simulink model "generic_IVS"  (R2024a)
settings: Solver=FixedStepDiscrete  StartTime=0.0  StopTime=inf  FixedStep=0.001  RelTol=1e-3
undefined symbols (not defined in the file): do_waypoints_tail_shifted_2, global_path_xy_second_test, pathXY, route1_waypoint, route1_waypoint_raw, route2_waypoint, route2_waypoint_raw, route3_waypoint, route3_waypoint_raw
libraries: CarMaker4SL x134, slpidlib x4, simulink x1
(part 5 of 5)

== matlab function generic_IVS/CarMaker/Subsystem/Final Project/Scenario 1/MATLAB Function ==
  settings: updateMethod=DISCRETE  sampleTime=1.0
  data: waypoints input; startIdx input; global_path_xy_dense output; must1 input; must2 input; goalIdx input; state input
% function global_path_xy_dense = make_global_path(waypoints, startIdx, must1, must2, goalIdx)
% %#codegen
% 
% N = size(waypoints,1);
% max_neighbors = 20;
% MAXLEN = 2000; % 충분히 크게
% 
% % --- via_nodes 처리 ---
% via_nodes = startIdx;
% if must1 ~= 0
%     via_nodes = [via_nodes, must1];
% end
% if must2 ~= 0
%     via_nodes = [via_nodes, must2];
% end
% via_nodes = [via_nodes, goalIdx];
% 
% % --- 진행방향 단위 벡터 계산 ---
% forward_vecs = zeros(N,2);
% for i = 1:N-1
%     v = waypoints(i+1,:) - waypoints(i,:);
%     vn = norm(v);
%     if vn > 1e-6
%         forward_vecs(i,:) = v / vn;
%     else
%         forward_vecs(i,:) = [1,0];
%     end
% end
% forward_vecs(N,:) = forward_vecs(N-1,:);
% 
% % --- 이웃 리스트 (고정 double array) ---
% neighborList = zeros(N, max_neighbors);
% neighborNum  = zeros(N,1);
% D_thresh = 5;
% 
% for i = 1:N
%     dists = sqrt(sum((waypoints - waypoints(i,:)).^2, 2));
%     candidateIdx = find(dists > 0 & dists < D_thresh);
% ncnt = 0;
% for j = 1:length(candidateIdx)
%     idx = candidateIdx(j);
%     vec = waypoints(idx,:) - waypoints(i,:);
%     vn2 = norm(vec);
%     if vn2 < 1e-6
%         continue;
%     end
%     vec = vec / vn2;
%     if dot(forward_vecs(i,:), vec) > 0
%         if ncnt < max_neighbors   % <--- 바꿔주세요!
%             ncnt = ncnt+1;
%             neighborList(i,ncnt) = idx;
%         end
%     end
% end
% neighborNum(i) = ncnt;
% end
% 
% % --- 전체 경로 연결 (via_nodes 순서대로, preallocation) ---
% full_path = zeros(N * (length(via_nodes)-1), 1);
% full_idx = 1;
% 
% for seg = 1:(length(via_nodes)-1)
%     sIdx = via_nodes(seg);
%     gIdx = via_nodes(seg+1);
% 
%     cameFrom = zeros(N,1);
%     gScore   = inf(N,1);
%     fScore   = inf(N,1);
% 
%     gScore(sIdx) = 0;
%     fScore(sIdx) = norm(waypoints(sIdx,:) - waypoints(gIdx,:));
%     openSet = zeros(N,1);
%     openSet(1) = sIdx;
%     openLen = 1;
% 
%     found = false;
%     while openLen > 0
%         fvalues = zeros(openLen,1);
%         for i = 1:openLen
%             fvalues(i) = fScore(openSet(i));
%         end
%         [~, minIdx] = min(fvalues);
%         current = openSet(minIdx);
%         if current == gIdx
%             found = true;
%             break;
%         end
%         if minIdx < openLen
%             openSet(minIdx:openLen-1) = openSet(minIdx+1:openLen);
%         end
%         openLen = openLen - 1;
% 
%         for nidx = 1:neighborNum(current)
%             neighbor = neighborList(current, nidx);
%             edge_cost = norm(waypoints(neighbor,:) - waypoints(current,:));
%             tentative_gScore = gScore(current) + edge_cost;
%             if tentative_gScore < gScore(neighbor)
%                 cameFrom(neighbor) = current;
%                 gScore(neighbor)   = tentative_gScore;
%                 fScore(neighbor)   = tentative_gScore + norm(waypoints(neighbor,:) - waypoints(gIdx,:));
%                 isin = false;
%                 for q = 1:openLen
%                     if openSet(q) == neighbor
%                         isin = true;
%                         break;
%                     end
%                 end
%                 if ~isin && openLen < N
%                     openLen = openLen+1;
%                     openSet(openLen) = neighbor;
%                 end
%             end
%         end
%     end
% 
%     if ~found
%         global_path_xy_dense = zeros(MAXLEN,2); % error 방지
%         return
%     end
% 
%     % --- 경로 추적 (preallocation) ---
%     MAX_PATH_LEN = N;
%     tmp_path = zeros(MAX_PATH_LEN, 1);
%     idx = 1;
%     curr = gIdx;
%     while curr ~= sIdx
%         tmp_path(idx) = curr;
%         curr = cameFrom(curr);
%         idx = idx + 1;
%         if idx > MAX_PATH_LEN
%             break;
%         end
%     end
%     tmp_path(idx) = sIdx;
%     path = tmp_path(idx:-1:1);
% 
%     if seg > 1
%         path = path(2:end);
%     end
% 
%     lenp = length(path);
%     full_path(full_idx : full_idx+lenp-1) = path;
%     full_idx = full_idx + lenp;
% end
% 
% full_path = full_path(1:full_idx-1);
% 
% % --- 경로 좌표 추출 ---
% global_path_xy = waypoints(full_path, :);
% 
% % --- 보간을 통한 촘촘한 경로 생성 ---
% diffs = diff(global_path_xy);
% seg_len = sqrt(sum(diffs.^2, 2));
% s = [0; cumsum(seg_len)];
% ds_interp = 0.5;
% if s(end) < ds_interp
%     interp_xy = global_path_xy;
% else
%     s_interp = (0:ds_interp:s(end))';
%     x_interp = interp1(s, global_path_xy(:,1), s_interp, 'linear');
%     y_interp = interp1(s, global_path_xy(:,2), s_interp, 'linear');
%     interp_xy = [x_interp, y_interp];
% end
% 
% global_path_xy_dense = zeros(MAXLEN,2);
% real_len = size(interp_xy,1);
% if real_len > MAXLEN
%     real_len = MAXLEN;
% end
% global_path_xy_dense(1:real_len,:) = interp_xy(1:real_len,:);
% end


function global_path_xy_dense = make_global_path_with_fsm_sfunc(waypoints, startIdx, must1, must2, goalIdx, state)
% Simulink에서 사용할 수 있도록 만든 FSM 기반 global path 생성 함수
% 입력:
%   waypoints [Nx2] double, startIdx/must1/must2/goalIdx/state: double scalar
% 출력:
%   global_path_xy_dense [MAXLEN x 2] double

%#codegen

MAXLEN = 2000;
N = size(waypoints,1);

persistent prev_goalIdx prev_full_path prev_flag

if isempty(prev_goalIdx)
    prev_goalIdx = goalIdx;
end
if isempty(prev_flag)
    prev_flag = 1; % default값. 반드시 0,1로만 동작
end

% Simulink 실행 시마다 state=0에서 "한 번만" 새 경로 생성
if state == 0
    startIdx_new = prev_goalIdx;
    must1_new = 0;
    must2_new = 0;
    goalIdx_new = 1565;

    % prev_flag가 1→0으로 바뀌는 순간 한 번만 실행
    if prev_flag ~= 0
        global_path_xy_dense = gen_global_path(waypoints, startIdx_new, must1_new, must2_new, goalIdx_new, N, MAXLEN);
        prev_full_path = global_path_xy_dense;
        prev_goalIdx = goalIdx_new;
    else
        % 이미 만든 경로 유지
        if isempty(prev_full_path)
            global_path_xy_dense = zeros(MAXLEN,2);
        else
            global_path_xy_dense = prev_full_path;
        end
    end
    prev_flag = 0;
else % state==1
    global_path_xy_dense = gen_global_path(waypoints, startIdx, must1, must2, goalIdx, N, MAXLEN);
    prev_full_path = global_path_xy_dense;
    prev_goalIdx = goalIdx;
    prev_flag = 1;
end

end

% ---- 내부 subfunction ----
function global_path_xy_dense = gen_global_path(waypoints, startIdx, must1, must2, goalIdx, N, MAXLEN)

max_neighbors = 20;
% --- via_nodes 처리 ---
via_nodes = startIdx;
if must1 ~= 0
    via_nodes = [via_nodes, must1];
end
if must2 ~= 0
    via_nodes = [via_nodes, must2];
end
via_nodes = [via_nodes, goalIdx];

% --- 진행방향 단위 벡터 계산 ---
forward_vecs = zeros(N,2);
for i = 1:N-1
    v = waypoints(i+1,:) - waypoints(i,:);
    vn = norm(v);
    if vn > 1e-6
        forward_vecs(i,:) = v / vn;
    else
        forward_vecs(i,:) = [1,0];
    end
end
forward_vecs(N,:) = forward_vecs(N-1,:);

% --- 이웃 리스트 ---
neighborList = zeros(N, max_neighbors);
neighborNum  = zeros(N,1);
D_thresh = 5;

for i = 1:N
    dists = sqrt(sum((waypoints - waypoints(i,:)).^2, 2));
    candidateIdx = find(dists > 0 & dists < D_thresh);
    ncnt = 0;
    for j = 1:length(candidateIdx)
        idx = candidateIdx(j);
        vec = waypoints(idx,:) - waypoints(i,:);
        vn2 = norm(vec);
        if vn2 < 1e-6
            continue;
        end
        vec = vec / vn2;
        if dot(forward_vecs(i,:), vec) > 0
            if ncnt < max_neighbors
                ncnt = ncnt+1;
                neighborList(i,ncnt) = idx;
            end
        end
    end
    neighborNum(i) = ncnt;
end

% --- 전체 경로 연결 (via_nodes 순서대로, preallocation) ---
full_path = zeros(N * (length(via_nodes)-1), 1);
full_idx = 1;

for seg = 1:(length(via_nodes)-1)
    sIdx = via_nodes(seg);
    gIdx = via_nodes(seg+1);

    cameFrom = zeros(N,1);
    gScore   = inf(N,1);
    fScore   = inf(N,1);

    gScore(sIdx) = 0;
    fScore(sIdx) = norm(waypoints(sIdx,:) - waypoints(gIdx,:));
    openSet = zeros(N,1);
    openSet(1) = sIdx;
    openLen = 1;

    found = false;
    while openLen > 0
        fvalues = zeros(openLen,1);
        for i = 1:openLen
            fvalues(i) = fScore(openSet(i));
        end
        [~, minIdx] = min(fvalues);
        current = openSet(minIdx);
        if current == gIdx
            found = true;
            break;
        end
        if minIdx < openLen
            openSet(minIdx:openLen-1) = openSet(minIdx+1:openLen);
        end
        openLen = openLen - 1;

        for nidx = 1:neighborNum(current)
            neighbor = neighborList(current, nidx);
            edge_cost = norm(waypoints(neighbor,:) - waypoints(current,:));
            tentative_gScore = gScore(current) + edge_cost;
            if tentative_gScore < gScore(neighbor)
                cameFrom(neighbor) = current;
                gScore(neighbor)   = tentative_gScore;
                fScore(neighbor)   = tentative_gScore + norm(waypoints(neighbor,:) - waypoints(gIdx,:));
                isin = false;
                for q = 1:openLen
                    if openSet(q) == neighbor
                        isin = true;
                        break;
                    end
                end
                if ~isin && openLen < N
                    openLen = openLen+1;
                    openSet(openLen) = neighbor;
                end
            end
        end
    end

    if ~found
        global_path_xy_dense = zeros(MAXLEN,2); % error 방지
        return
    end

    % --- 경로 추적 (preallocation) ---
    MAX_PATH_LEN = N;
    tmp_path = zeros(MAX_PATH_LEN, 1);
    idx = 1;
    curr = gIdx;
    while curr ~= sIdx
        tmp_path(idx) = curr;
        curr = cameFrom(curr);
        idx = idx + 1;
        if idx > MAX_PATH_LEN
            break;
        end
    end
    tmp_path(idx) = sIdx;
    path = tmp_path(idx:-1:1);

    if seg > 1
        path = path(2:end);
    end

    lenp = length(path);
    full_path(full_idx : full_idx+lenp-1) = path;
    full_idx = full_idx + lenp;
end

full_path = full_path(1:full_idx-1);

% --- 경로 좌표 추출 ---
global_path_xy = waypoints(full_path, :);

% --- 보간을 통한 촘촘한 경로 생성 ---
diffs = diff(global_path_xy);
seg_len = sqrt(sum(diffs.^2, 2));
s = [0; cumsum(seg_len)];
ds_interp = 0.5;
if s(end) < ds_interp
    interp_xy = global_path_xy;
else
    s_interp = (0:ds_interp:s(end))';
    x_interp = interp1(s, global_path_xy(:,1), s_interp, 'linear');
    y_interp = interp1(s, global_path_xy(:,2), s_interp, 'linear');
    interp_xy = [x_interp, y_interp];
end

global_path_xy_dense = zeros(MAXLEN,2);
real_len = size(interp_xy,1);
if real_len > MAXLEN
    real_len = MAXLEN;
end
global_path_xy_dense(1:real_len,:) = interp_xy(1:real_len,:);
end

== matlab function generic_IVS/CarMaker/Subsystem/Final Project/Scenario 1/MATLAB Function1 ==
  data: u1 input; target_speed_out output; u2 input; target_speed_in input
% function y = and_logic_latch_permanent(u1, u2)
% %#codegen
% persistent latch;
% if isempty(latch)
%     latch = 0;
% end
% 
% % 정지 조건에 한 번이라도 들어가면 latch=1이 되고, 이후엔 절대 복귀하지 않음
% if (u1 > 5) && (u1 < 6) && (u2 > -38) && (u2 < -35)
%     latch = 1;
% end
% 
% y = latch;
% end



function target_speed_out = and_logic_latch_speed(u1, u2, target_speed_in)
%#codegen
persistent latch;
if isempty(latch)
    latch = 0;
end

% 정지 조건에 한 번이라도 들어가면 latch=1이 되고, 이후엔 절대 복귀하지 않음
if (u1 > 5) && (u1 < 6) && (u2 > -38) && (u2 < -35)
    latch = 1;
end

if latch == 1
    target_speed_out = 0;
else
    target_speed_out = target_speed_in;
end
end

== matlab function generic_IVS/CarMaker/Subsystem/Final Project/Scenario 1/MATLAB Function2 ==
  settings: updateMethod=DISCRETE  sampleTime=0.05
  data: waypoints_x input; waypoints_y input; X_ego input; Y_ego input; head input; steering_angle output; goal_pose input; speed output; x_local output; y_local output
function [steering_angle, speed, x_local, y_local] = ...
    global_to_local_waypoints(waypoints_x, waypoints_y, ...
                              X_ego, Y_ego, head, goal_pose)
%#codegen

    %% 파라미터
    stop_threshold = 4.5;
    heading_align_threshold = 10.0;
    v_base = 3.0;          % 기본 속도 [m/s]
    v_min = 1.5;           % 최소 속도
    v_max = 5.0;           % 최대 속도

    %% 출력 초기화
    x_local = 0.0;
    y_local = 0.0;
    steering_angle = 0;
    speed = v_base;

    %% 목표점까지 거리 계산
    goal_dist = norm([X_ego - goal_pose(1), Y_ego - goal_pose(2)]);

    %% 1) 정지 조건
    if goal_dist < stop_threshold
        speed = 0;
        steering_angle = 0;
        return;
    end

    %% 2) 헤딩 정렬 조건
    if goal_dist < heading_align_threshold
        heading_error = wrapToPi(pi/2 - head);  % 90도 방향으로 정렬
        steering_angle = atan2(2 * 2.9 * sin(heading_error), goal_dist + 1e-3);
        speed = 3;
        return;
    end

    %% 3) 유효한 웨이포인트 필터링
    valid_idx = ~isnan(waypoints_x) & ~isnan(waypoints_y);
    x_wp = waypoints_x(valid_idx);
    y_wp = waypoints_y(valid_idx);
    N = numel(x_wp);
    if N == 0
        speed = 0;
        return;
    end

    %% 4) 가장 가까운 포인트의 로컬 좌표 저장
    distances = sqrt((x_wp - X_ego).^2 + (y_wp - Y_ego).^2);
    [~, idx_closest] = min(distances);
    dx = x_wp(idx_closest) - X_ego;
    dy = y_wp(idx_closest) - Y_ego;
    x_local = dx * cos(-head) - dy * sin(-head);
    y_local = dx * sin(-head) + dy * cos(-head);

    %% 5) Pure Pursuit 조향각 계산
    [steering_angle, ~] = pure_pursuit(x_wp, y_wp, [X_ego, Y_ego], head);

    %% 6) 속도 고정 또는 조정 (간단히 유지)
    speed = max(v_min, min(v_base, v_max));
end

%% ===== Pure Pursuit 함수 =====
function [steering_angle, start_idx] = pure_pursuit(waypoints_x, waypoints_y, vehicle_position, head)
    persistent last_target_idx;
    if isempty(last_target_idx)
        last_target_idx = 1;
    end

    WHEEL_BASE = 2.9;
    lookahead_dist = 3.0;
    num_points = length(waypoints_x);

    x_ego = vehicle_position(1);
    y_ego = vehicle_position(2);
    local_waypoints = zeros(num_points, 2);

    for i = 1:num_points
        dx = waypoints_x(i) - x_ego;
        dy = waypoints_y(i) - y_ego;
        local_x = dx * cos(-head) - dy * sin(-head);
        local_y = dx * sin(-head) + dy * cos(-head);
        local_waypoints(i, :) = [local_x, local_y];
    end    

    distances_to_waypoints = sqrt((waypoints_x - x_ego).^2 + (waypoints_y - y_ego).^2);
    [~, closest_idx] = min(distances_to_waypoints);
    start_idx = max(last_target_idx, closest_idx);

    target_idx = -1;
    final_ld = 0;
    for i = start_idx:num_points
        dist = norm(local_waypoints(i, :));
        if dist > lookahead_dist && local_waypoints(i, 1) > 0
            target_idx = i;
            final_ld = dist;
            break;
        end
    end

    if target_idx == -1
        for i = 1:start_idx-1
            dist = norm(local_waypoints(i, :));
            if dist > lookahead_dist && local_waypoints(i, 1) > 0
                target_idx = i;
                final_ld = dist;
                break;
            end
        end
    end

    if target_idx == -1
        steering_angle = 0;
        return;
    end

    target_point = local_waypoints(target_idx, :);
    alpha = atan2(target_point(2), target_point(1));
    alpha = wrapToPi(alpha);
    final_ld = min(max(final_ld, 2.0), 20.0);

    steering_angle = atan2(2 * WHEEL_BASE * sin(alpha), final_ld);
    last_target_idx = target_idx;
end

%% ===== 각도 wrap 함수 =====
function angle = wrapToPi(theta)
    angle = mod(theta + pi, 2*pi) - pi;
end

== matlab function generic_IVS/CarMaker/Subsystem/Final Project/Scenario 1/MATLAB Function5 ==
  settings: updateMethod=DISCRETE  sampleTime=0.05
  data: map_boundary input; mapMatrix output size=[1000, 1000]; traffic_info input
%% ======== generate_map_ ======== Ver 2025-05-17 10:40
function mapMatrix  = generate_map_(map_boundary, traffic_info)
    %변수설정
    resolution = 0.05;
    traffic_info_mat = reshape(traffic_info(1:5*21), 5, []).';
    x_values = map_boundary(1:2:end);
    y_values = map_boundary(2:2:end);
    N = size(traffic_info_mat,1);
    x_min = min(x_values);  x_max = max(x_values);
    y_min = min(y_values);  y_max = max(y_values);
    x_size = ceil((x_max-x_min)/resolution);
    y_size = ceil((y_max-y_min)/resolution);
    
    
    mapMatrix = zeros(y_size, x_size); %출력코드
    
    for i = 1:N
        x_c = traffic_info_mat(i, 1);
        y_c = traffic_info_mat(i, 2);
        yaw = traffic_info_mat(i, 3);
        length = traffic_info_mat(i, 4);
        width = traffic_info_mat(i, 5);
        
        if yaw == -1.57079628
            yaw = -pi/2;
        elseif yaw == 1.57079628
            yaw = pi/2;
        end

        dx = length/2;  dy = width/2;
        local = [-dx,-dy; dx,-dy; dx,dy; -dx,dy];
        R = [cos(yaw), -sin(yaw); sin(yaw), cos(yaw)];
        rotated = (R*local')';
        forward_vec = [cos(yaw), sin(yaw)];
        side_vec    = [-sin(yaw), cos(yaw)];
        if yaw == -pi/2
            center = [x_c, y_c] + (length/2)*forward_vec + (width/2)*side_vec;
        else
            center = [x_c, y_c] + (length/2)*forward_vec - (width/2)*side_vec;
        end
        corners = rotated + center;
        x_idx = (corners(:,1)-x_min)/resolution + 1;
        y_idx = (y_max-corners(:,2))/resolution + 1;
        mask = poly2mask(x_idx, y_idx, y_size, x_size);
        mapMatrix(mask) = 1;
    end
end

== matlab function generic_IVS/CarMaker/Subsystem/Final Project/Scenario 1/MATLAB Function6 ==
  settings: updateMethod=DISCRETE  sampleTime=0.05
  data: map input; x_path output; startPose input; goalPose input; y_path output; mapboundary input
function [x_path, y_path] = rrt_star_planner(map, startPose, goalPose, mapboundary)
    %% ===== Persistent 저장 =====
    persistent path_initialized x_path_cached y_path_cached nPath_cached
    maxPathLength = 500;
    resolution = 0.05;

    if isempty(path_initialized)
        path_initialized = false;
        x_path_cached = zeros(maxPathLength, 1);
        y_path_cached = zeros(maxPathLength, 1);
        nPath_cached = 1;
    end

    % if path_initialized
    %     x_path = x_path_cached(1:nPath_cached);
    %     y_path = y_path_cached(1:nPath_cached);
    %     return;
    % end
    %% global_y가 안 떠서 수정함.
    if path_initialized && nPath_cached >= 2
        x_path = x_path_cached(1:nPath_cached);
        y_path = y_path_cached(1:nPath_cached);
        return;
    elseif path_initialized
        % 캐시에 저장된 경로가 너무 짧으면 의미 없는 0벡터라도 반환
        x_path = zeros(2,1);
        y_path = zeros(2,1);
        return;
    end

    %% 설정
    visualize      = false;
    maxIter        = 5000;
    stepSize       = 2;
    goalSampleRate = 0.1;
    successDistTh  = 5;
    collisionRes   = 0.5;
    searchRadius   = 10;
    safetyDist     = 0;

    %% 바운더리 기반 인덱스 변환용 파라미터
    x_values = mapboundary(1:2:end);
    y_values = mapboundary(2:2:end);
    x_min = min(x_values);
    y_max = max(y_values);

    %% 실좌표 → 인덱스 변환
    toGrid = @(x, y) [(x - x_min)/resolution +  1, (y_max - y)/resolution + 1];

    start_grid = toGrid(startPose(1), startPose(2));
    goal_grid  = toGrid(goalPose(1), goalPose(2));

    %% 트리 초기화 (모든 노드는 인덱스 좌표로 유지)
    nodes = struct('x', start_grid(1), 'y', start_grid(2), ...
                   'parent', 0, 'cost', 0);

    %% 경로 및 출력 초기화
    path   = struct('x', {}, 'y', {}, 'parent', {}, 'cost', {});
    x_path = zeros(maxPathLength, 1);
    y_path = zeros(maxPathLength, 1);

    %% RRT* 메인 루프 (모든 연산 인덱스 기반)
    for iter = 1:maxIter
        if rand < goalSampleRate
            xr = goal_grid;
        else
            xr = [randi([1, size(map,2)]), randi([1, size(map,1)])];
        end

        [nearestIdx, nearXY] = findNearest(nodes, xr);
        theta = atan2(xr(2)-nearXY(2), xr(1)-nearXY(1));
        newXY = nearXY + stepSize * [cos(theta), sin(theta)];

        if isCollision(newXY, map) || ...
           isPathCollision(nearXY, newXY, map, collisionRes) || ...
           isNearObstacle(newXY, map, safetyDist / resolution)
            continue;
        end

        nearIdxs = findNearNodes(nodes, newXY, searchRadius);
        minCost   = nodes(nearestIdx).cost + norm(newXY - nearXY);
        minParent = nearestIdx;

        for idx = 1:numel(nearIdxs)
            iNode = nearIdxs(idx);
            pxy   = [nodes(iNode).x, nodes(iNode).y];
            if ~isPathCollision(pxy, newXY, map, collisionRes)
                c = nodes(iNode).cost + norm(newXY - pxy);
                if c < minCost
                    minCost   = c;
                    minParent = iNode;
                end
            end
        end

        newNode = struct('x', newXY(1), 'y', newXY(2), ...
                         'parent', minParent, 'cost', minCost);
        nodes(end+1) = newNode;
        newIdx       = numel(nodes);

        for idx = 1:numel(nearIdxs)
            iNode = nearIdxs(idx);
            pxy   = [nodes(iNode).x, nodes(iNode).y];
            c     = newNode.cost + norm([newNode.x, newNode.y] - pxy);
            if c < nodes(iNode).cost && ...
               ~isPathCollision([newNode.x,newNode.y], pxy, map, collisionRes)
                nodes(iNode).parent = newIdx;
                nodes(iNode).cost   = c;
            end
        end

        if visualize
            plot([nodes(newNode.parent).x, newNode.x], ...
                 [nodes(newNode.parent).y, newNode.y], '-r');
            hold on;
        end

        if norm(newXY - goal_grid) < successDistTh
            if visualize, disp('[-] GOAL REACHED'); end
            path = backtrace(nodes, newIdx);
            break;
        end
    end

    %% 결과 경로 반환 (인덱스 → 실좌표로 역변환)
    nPath = min(numel(path), maxPathLength);
    x_path_cached = zeros(maxPathLength, 1);
    y_path_cached = zeros(maxPathLength, 1);
    for k = 1:nPath
        x_path_cached(k) = (path(k).x - 1) * resolution + x_min;
        y_path_cached(k) = y_max - (path(k).y - 1) * resolution;
    end

    nPath_cached = nPath;
    path_initialized = true;

    %% === Lightweight Smoothing for Simulink Compatibility ===
    smooth_window = 15;  % 홀수 추천
    if nPath >= smooth_window
        x = x_path_cached(1:nPath);
        y = y_path_cached(1:nPath);

        x_smooth = movmean(x, smooth_window);
        y_smooth = movmean(y, smooth_window);

        % 재샘플링 (고정된 개수로)
        smoothN = 100;
        idx_original = linspace(1, numel(x_smooth), smoothN);
        x_path = interp1(1:numel(x_smooth), x_smooth, idx_original, 'linear')';
        y_path = interp1(1:numel(y_smooth), y_smooth, idx_original, 'linear')';
    else
        x_path = x_path_cached(1:nPath);
        y_path = y_path_cached(1:nPath);
    end


end

%% ======= 서브 함수들 =======

function [idx, xy] = findNearest(nodes, sampleXY)
    d = arrayfun(@(n) hypot(n.x - sampleXY(1), n.y - sampleXY(2)), nodes);
    [~, idx] = min(d);
    xy = [nodes(idx).x, nodes(idx).y];
end

function nearIdxs = findNearNodes(nodes, pos, radius)
    maxNodes = 1000;
    nearIdxs = zeros(1, maxNodes);
    count = 0;
    for i = 1:numel(nodes)
        if hypot(nodes(i).x - pos(1), nodes(i).y - pos(2)) <= radius
            count = count + 1;
            nearIdxs(count) = i;
        end
    end
    nearIdxs = nearIdxs(1:count);
end

function flag = isCollision(pt, map)
    x = round(pt(1)); y = round(pt(2));
    flag = x < 1 || x > size(map,2) || y < 1 || y > size(map,1) || map(y,x) == 1;
end

function flag = isPathCollision(p1, p2, map, step)
    dist = norm(p2 - p1);
    N = max(1, ceil(dist / step));
    flag = false;
    for i = 0:N
        pt = p1 + (p2 - p1) * (i / N);
        if isCollision(pt, map)
            flag = true; return;
        end
    end
end

function flag = isNearObstacle(pt, map, safeDist)
    x0 = round(pt(1)); y0 = round(pt(2));
    r  = ceil(safeDist);
    [X, Y] = meshgrid((x0 - r):(x0 + r), (y0 - r):(y0 + r));
    D2 = (X - pt(1)).^2 + (Y - pt(2)).^2;
    mask = D2 <= safeDist^2;
    X = X(mask); Y = Y(mask);
    valid = X >= 1 & X <= size(map,2) & Y >= 1 & Y <= size(map,1);
    flag  = any(map(sub2ind(size(map), Y(valid), X(valid))) == 1);
end

function path = backtrace(nodes, idx)
    maxPathLen = 500;
    dummyNode = struct('x', 0, 'y', 0, 'parent', 0, 'cost', 0);
    path = repmat(dummyNode, maxPathLen, 1);
    count = 0;
    while idx ~= 0 && count < maxPathLen
        count = count + 1;
        path(count) = nodes(idx);
        idx = nodes(idx).parent;
    end
    path = path(count:-1:1);
end

== stateflow chart generic_IVS/CarMaker/Subsystem/Day3/Chart ==
  (default) -> (junction 1)
  (junction 1) -> (junction 3) [order 1] : [i<99]
      | {i = i + 1;}
  (junction 1) -> (junction 7) [order 2] : {i=0;}
  (junction 3) -> (junction 5)
  (junction 5) -> (junction 7)
  (junction 7) -> (junction 10)
  (junction 10) -> (junction 12) [order 1] : [rem(i,50) == 0]
      | {do_Logic;}
  (junction 10) -> (junction 18) [order 2]
  (junction 12) -> (junction 16)
  (junction 16) -> (junction 18)
  (junction 18) -> (junction 21)
  data: i local =0
  events: do_Logic output FUNCTION_CALL_EVENT
